simulink model "model"  (R2022b)
settings: Solver=ode3  StartTime=0.0  StopTime=Tmdl  FixedStep=T/1000  RelTol=1e-3
values from neighbouring files (symbols this model uses):
  K1 = 85    [data.mat]
  K2 = 70    [data.mat]
  K3 = 0.02    [data.mat]
  T = 0.005    [data.mat]
  T1 = 0.09    [data.mat]
  T2 = 0.1    [data.mat]
settings Model: Creator=R1505-We2-2-Stud  LastModifiedBy=R1505-We2-2-Stud

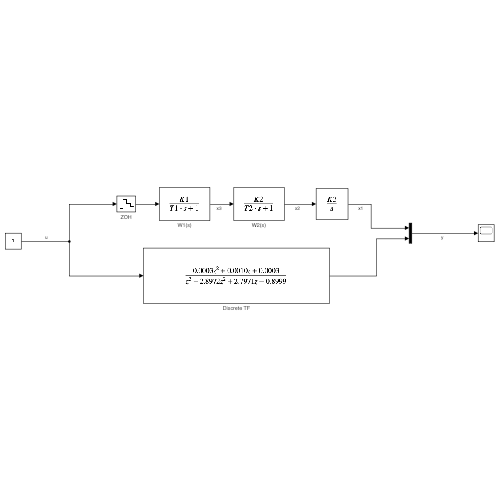
[thumbnail: Simulink's stored preview of the top-level diagram]
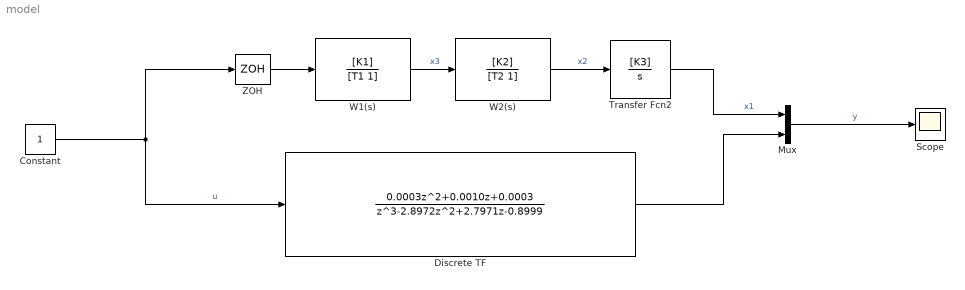
== system model ==
  Constant : Constant
  Discrete TF : DiscreteTransferFcn  Numerator=[0.0003 0.0010 0.0003]  Denominator=[1 -2.8972 2.7971 -0.8999]  SampleTime=T
  Mux : Mux  Inputs=2
  Scope : Scope
  Transfer Fcn2 : TransferFcn  Numerator=[K3]  Denominator=[1 0]
  W1(s) : TransferFcn  Numerator=[K1]  Denominator=[T1 1]
  W2(s) : TransferFcn  Numerator=[K2]  Denominator=[T2 1]
  ZOH : ZeroOrderHold  SampleTime=-1
  wires:
  W1(s)/1 -> W2(s)/1  "x3"
  W2(s)/1 -> Transfer Fcn2/1  "x2"
  ZOH/1 -> W1(s)/1
  Transfer Fcn2/1 -> Mux/1  "x1"
  Discrete TF/1 -> Mux/2
  Constant/1 -> ZOH/1, Discrete TF/1  "u"
  Mux/1 -> Scope/1  "y"
